simulink model "Car_with_active_suspension_controller"  (R2024b)
settings: Solver=ode45  StartTime=0  StopTime=45  FixedStep=0.001  RelTol=1e-3  AbsTol=1e-6
libraries: simulink_extras x4, Solver_SF x1
settings Model: Creator=ywata  LastModifiedBy=ASUS
settings SolverCC: AutoScaleAbsTol=off  AlgebraicLoopSolver=TrustRegion
settings DataIOCC: SaveFormat=Array  SignalLoggingSaveFormat=ModelDataLogs  ReturnWorkspaceOutputs=off  SignalLoggingName=sigsOut
settings OptimizationCC: BooleanDataType=off  LifeSpan=inf
settings DebuggingCC: SaveWithParameterizedLinksMsg=none  UnderspecifiedInitializationDetection=Classic  MergeDetectMultiDrivingBlocksExec=none  SignalResolutionControl=TryResolveAllWithWarning  MultiTaskDSMMsg=warning  MultiTaskCondExecSysMsg=none  FcnCallInpInsideContextMsg=warning  UnconnectedInputMsg=warning  UnconnectedOutputMsg=warning  UnconnectedLineMsg=warning  StateNameClashWarn=warning  SFUnexpectedBacktrackingDiag=warning  SFNoUnconditionalDefaultTransitionDiag=warning  SFExecutionAtInitializationDiag=none  ArithmeticOperatorsInVariantConditions=warning
settings HardwareCC: ProdBitPerPointer=32  ProdBitPerSizeT=32  ProdBitPerPtrDiffT=32  ProdLargestAtomicFloat=None  ProdIntDivRoundTo=Undefined  ProdEndianess=Unspecified  ProdWordSize=32  ProdHWDeviceType=32-bit Generic  TargetUnknown=on
settings ModelReferenceCC: PropagateSignalLabelsOutOfModel=off
settings RTWCC: TemplateMakefile=grt_vc.tmf  GPUComputeCapability=3.5
settings CodeAppCC: StateflowObjectComments=on
settings GRTTargetCC: TargetLangStandard=C89/C90 (ANSI)  CombineOutputUpdateFcns=off  GRTInterface=on
settings ConfigComp: CovMetricSettings=dw  CovSaveCumulativeToWorkspaceVar=on  CovSaveSingleToWorkspaceVar=on

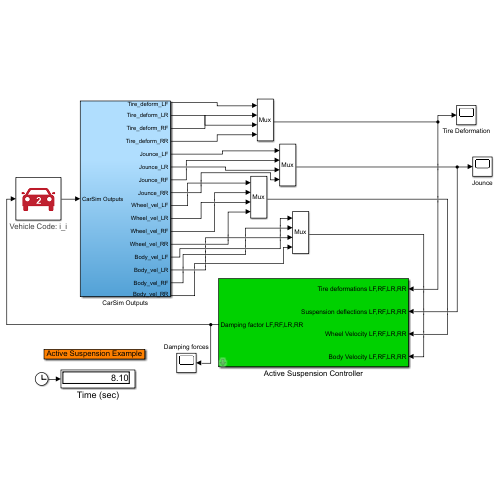
[thumbnail: Simulink's stored preview of the top-level diagram]
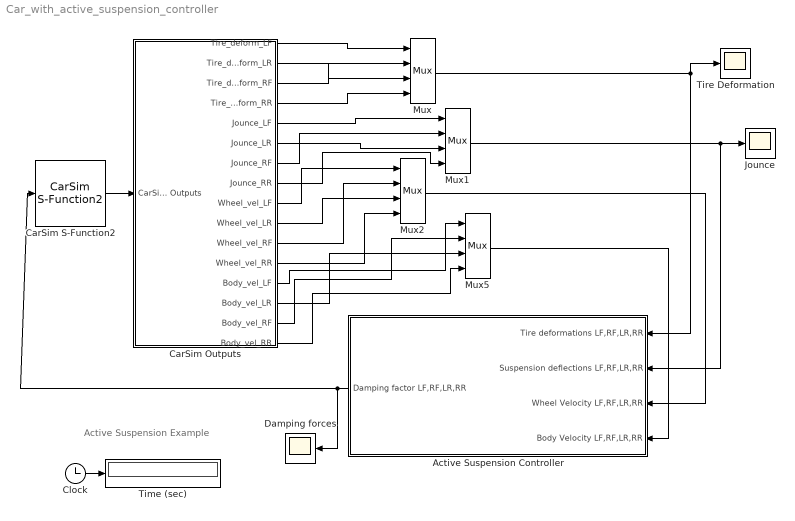
== system Car_with_active_suspension_controller ==
  note: Active Suspension Example
  Active Suspension Controller : Subsystem  mask{K1=-14184, K2=8624, K3=1088, K4=-2504, SP_F=65000, SP_R=52000, GAIN1=1, GAIN2=2.5, UPLIM=40000, LWLIM=10}
      mask prompts: K1 "Optimal control gain, K1"; K2 "Optimal control gain, K2"; K3 "Optimal control gain, K3"; K4 "Optimal control gain, K4"; SP_F "Spring stiffness (front)  (N/m)"; SP_R "Spring stiffness (rear)  (N/m)"; GAIN1 "Gain 1"; GAIN2 "Gain 2"; UPLIM "Variable damper upper limit (N-s/m)"; LWLIM "Variable damper lower limit (N-s/m)"
  CarSim Outputs : Subsystem
  CarSim S-Function2 : Solver_SF/CarSim S-Function2  Priority=1  VehicleCode=i_i  SIMFILE=simfile.sim
      settings: AttributesFormatString=Vehicle Code: %<VehicleCode>  SourceProductName=CarSim S-Function
  Clock : Clock
  Damping forces : Scope
  Jounce : Scope
  Mux{,1..2,5} (4 alike) : Mux
  Time (sec) : Display
      settings: Format=bank  Decimation=100
  Tire Deformation : Scope
  wires:
  Mux2/1 -> Active Suspension Controller/3(Wheel Velocity LF,RF,LR,RR)
  Mux5/1 -> Active Suspension Controller/4(Body Velocity LF,RF,LR,RR)
  Mux/1 -> Active Suspension Controller/1(Tire deformations LF,RF,LR,RR), Tire Deformation/1
  Mux1/1 -> Jounce/1, Active Suspension Controller/2(Suspension deflections LF,RF,LR,RR)
  CarSim Outputs/1(Tire_deform_LF) -> Mux/1
  CarSim Outputs/2(Tire_deform_LR) -> Mux/3
  CarSim Outputs/3(Tire_deform_RF) -> Mux/2
  CarSim Outputs/5(Jounce_LF) -> Mux1/1
  CarSim Outputs/6(Jounce_LR) -> Mux1/3
  CarSim Outputs/7(Jounce_RF) -> Mux1/2
  CarSim Outputs/8(Jounce_RR) -> Mux1/4
  CarSim Outputs/9(Wheel_vel_LF) -> Mux2/1
  CarSim Outputs/10(Wheel_vel_LR) -> Mux2/3
  CarSim Outputs/11(Wheel_vel_RF) -> Mux2/2
  CarSim Outputs/12(Wheel_vel_RR) -> Mux2/4
  CarSim Outputs/13(Body_vel_LF) -> Mux5/1
  CarSim Outputs/14(Body_vel_LR) -> Mux5/3
  CarSim Outputs/15(Body_vel_RF) -> Mux5/2
  CarSim Outputs/16(Body_vel_RR) -> Mux5/4
  CarSim S-Function2/1 -> CarSim Outputs/1(CarSim Outputs)
  CarSim Outputs/4(Tire_deform_RR) -> Mux/4
  Clock/1 -> Time (sec)/1
  Active Suspension Controller/1(Damping factor LF,RF,LR,RR) -> Damping forces/1, CarSim S-Function2/1

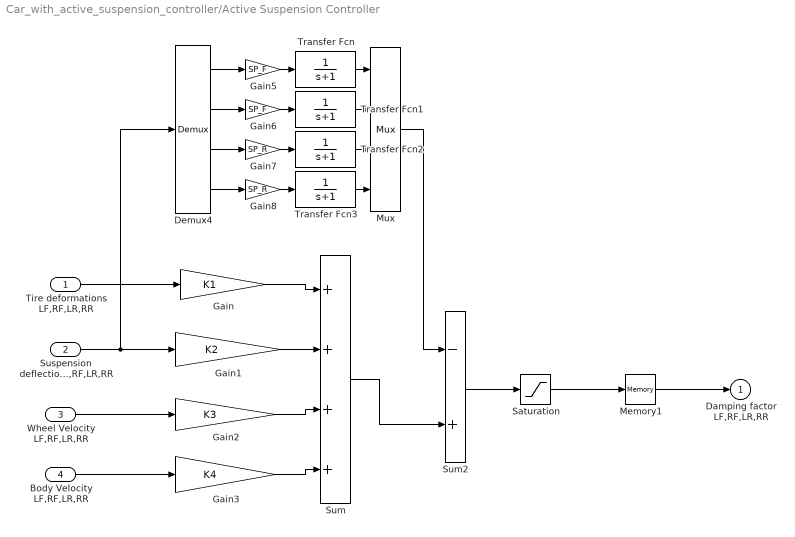
== system Car_with_active_suspension_controller/Active Suspension Controller ==
  Tire deformations LF,RF,LR,RR : Inport
  Suspension deflections LF,RF,LR,RR : Inport  Port=2
  Wheel Velocity LF,RF,LR,RR : Inport  Port=3
  Body Velocity LF,RF,LR,RR : Inport  Port=4
  Demux4 : Demux
      settings: DisplayOption=none
  Gain : Gain  Gain=K1  SaturateOnIntegerOverflow=on  OutDataTypeStr=Inherit: Same as input  ParamDataTypeStr=Inherit: Same as input
  Gain1 : Gain  Gain=K2  SaturateOnIntegerOverflow=on  OutDataTypeStr=Inherit: Same as input  ParamDataTypeStr=Inherit: Same as input
  Gain2 : Gain  Gain=K3  SaturateOnIntegerOverflow=on  OutDataTypeStr=Inherit: Same as input  ParamDataTypeStr=Inherit: Same as input
  Gain3 : Gain  Gain=K4  SaturateOnIntegerOverflow=on  OutDataTypeStr=Inherit: Same as input  ParamDataTypeStr=Inherit: Same as input
  Gain5 : Gain  Gain=SP_F  SaturateOnIntegerOverflow=on  OutDataTypeStr=Inherit: Same as input  ParamDataTypeStr=Inherit: Same as input
  Gain6 : Gain  Gain=SP_F  SaturateOnIntegerOverflow=on  OutDataTypeStr=Inherit: Same as input  ParamDataTypeStr=Inherit: Same as input
  Gain7 : Gain  Gain=SP_R  SaturateOnIntegerOverflow=on  OutDataTypeStr=Inherit: Same as input  ParamDataTypeStr=Inherit: Same as input
  Gain8 : Gain  Gain=SP_R  SaturateOnIntegerOverflow=on  OutDataTypeStr=Inherit: Same as input  ParamDataTypeStr=Inherit: Same as input
  Memory1 : Memory
  Mux : Mux
  Saturation : Saturate  UpperLimit=UPLIM  LowerLimit=LWLIM
  Sum : Sum  Inputs=++++  InputSameDT=on  SaturateOnIntegerOverflow=on  OutDataTypeStr=Inherit: Same as first input
  Sum2 : Sum  Inputs=-+  InputSameDT=on  SaturateOnIntegerOverflow=on  OutDataTypeStr=Inherit: Same as first input
  Transfer Fcn{,1..3} (4 alike) : TransferFcn  Denominator=[1 1]
  Damping factor LF,RF,LR,RR : Outport  InitialOutput=0
  wires:
  Tire deformations LF,RF,LR,RR/1 -> Gain/1
  Gain/1 -> Sum/1
  Gain1/1 -> Sum/2
  Gain2/1 -> Sum/3
  Gain3/1 -> Sum/4
  Sum2/1 -> Saturation/1
  Body Velocity LF,RF,LR,RR/1 -> Gain3/1
  Wheel Velocity LF,RF,LR,RR/1 -> Gain2/1
  Saturation/1 -> Memory1/1
  Memory1/1 -> Damping factor LF,RF,LR,RR/1
  Suspension deflections LF,RF,LR,RR/1 -> Gain1/1, Demux4/1
  Demux4/1 -> Gain5/1
  Demux4/2 -> Gain6/1
  Demux4/3 -> Gain7/1
  Demux4/4 -> Gain8/1
  Sum/1 -> Sum2/2
  Mux/1 -> Sum2/1
  Gain8/1 -> Transfer Fcn3/1
  Transfer Fcn3/1 -> Mux/4
  Gain7/1 -> Transfer Fcn2/1
  Transfer Fcn2/1 -> Mux/3
  Gain6/1 -> Transfer Fcn1/1
  Transfer Fcn1/1 -> Mux/2
  Gain5/1 -> Transfer Fcn/1
  Transfer Fcn/1 -> Mux/1

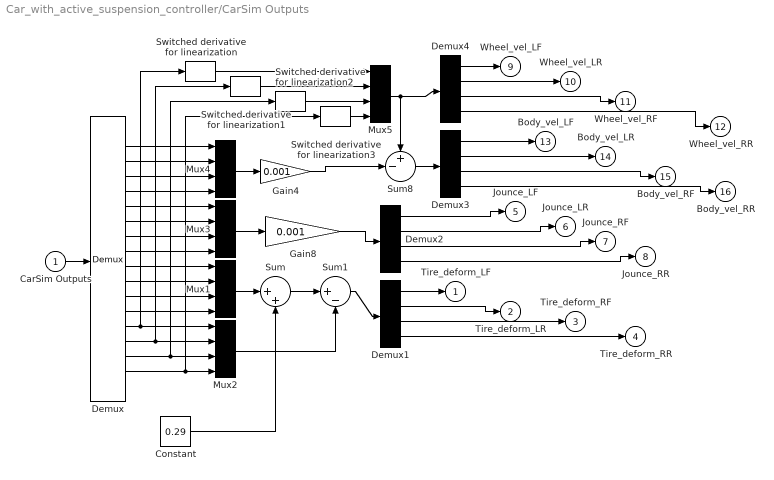
== system Car_with_active_suspension_controller/CarSim Outputs ==
  CarSim Outputs : Inport
  Constant : Constant  Value=0.29
  Demux : Demux  Outputs=16
      settings: DisplayOption=none
  Demux{1..4} (4 alike) : Demux
      settings: DisplayOption=none
  Gain4 : Gain  Gain=0.001  SaturateOnIntegerOverflow=on  OutDataTypeStr=Inherit: Same as input  ParamDataTypeStr=Inherit: Same as input
  Gain8 : Gain  Gain=0.001  SaturateOnIntegerOverflow=on  OutDataTypeStr=Inherit: Same as input  ParamDataTypeStr=Inherit: Same as input
  Mux{1..5} (5 alike) : Mux
  Sum : Sum  Inputs=|++  InputSameDT=on  SaturateOnIntegerOverflow=on  OutDataTypeStr=Inherit: Same as first input
  Sum1 : Sum  Inputs=|+-  InputSameDT=on  SaturateOnIntegerOverflow=on  OutDataTypeStr=Inherit: Same as first input
  Sum8 : Sum  Inputs=+-|  InputSameDT=on  SaturateOnIntegerOverflow=on  OutDataTypeStr=Inherit: Same as first input
  Switched derivative for linearization{,1..3} (4 alike) : simulink_extras/Linearization/Switched derivative for linearization  switchVal=0  derivConst=100
  Tire_deform_LF : Outport  InitialOutput=0
  Tire_deform_LR : Outport  Port=2  InitialOutput=0
  Tire_deform_RF : Outport  Port=3  InitialOutput=0
  Tire_deform_RR : Outport  Port=4  InitialOutput=0
  Jounce_LF : Outport  Port=5  InitialOutput=0
  Jounce_LR : Outport  Port=6  InitialOutput=0
  Jounce_RF : Outport  Port=7  InitialOutput=0
  Jounce_RR : Outport  Port=8  InitialOutput=0
  Wheel_vel_LF : Outport  Port=9  InitialOutput=0
  Wheel_vel_LR : Outport  Port=10  InitialOutput=0
  Wheel_vel_RF : Outport  Port=11  InitialOutput=0
  Wheel_vel_RR : Outport  Port=12  InitialOutput=0
  Body_vel_LF : Outport  Port=13  InitialOutput=0
  Body_vel_LR : Outport  Port=14  InitialOutput=0
  Body_vel_RF : Outport  Port=15  InitialOutput=0
  Body_vel_RR : Outport  Port=16  InitialOutput=0
  wires:
  Sum/1 -> Sum1/1
  Mux1/1 -> Sum/1
  Constant/1 -> Sum/2
  Mux2/1 -> Sum1/2
  Sum1/1 -> Demux1/1
  Demux1/1 -> Tire_deform_LF/1
  Demux1/2 -> Tire_deform_LR/1
  Demux1/3 -> Tire_deform_RF/1
  Demux1/4 -> Tire_deform_RR/1
  Mux3/1 -> Gain8/1
  Gain8/1 -> Demux2/1
  Demux2/1 -> Jounce_LF/1
  Demux2/2 -> Jounce_LR/1
  Demux2/3 -> Jounce_RF/1
  Demux2/4 -> Jounce_RR/1
  Sum8/1 -> Demux3/1
  Demux3/1 -> Body_vel_LF/1
  Demux3/2 -> Body_vel_LR/1
  Demux3/3 -> Body_vel_RF/1
  Demux3/4 -> Body_vel_RR/1
  Demux4/1 -> Wheel_vel_LF/1
  Demux4/2 -> Wheel_vel_LR/1
  Demux4/3 -> Wheel_vel_RF/1
  Demux4/4 -> Wheel_vel_RR/1
  Mux4/1 -> Gain4/1
  Gain4/1 -> Sum8/2
  Demux/12 -> Mux1/4
  Demux/11 -> Mux1/3
  Demux/10 -> Mux1/2
  Demux/9 -> Mux1/1
  Demux/8 -> Mux3/4
  Demux/7 -> Mux3/3
  Demux/6 -> Mux3/2
  Demux/5 -> Mux3/1
  Demux/4 -> Mux4/4
  Demux/3 -> Mux4/3
  Demux/2 -> Mux4/2
  Demux/1 -> Mux4/1
  Demux/13 -> Mux2/1, Switched derivative for linearization/1
  Demux/14 -> Mux2/2, Switched derivative for linearization1/1
  Demux/15 -> Mux2/3, Switched derivative for linearization2/1
  Demux/16 -> Mux2/4, Switched derivative for linearization3/1
  Switched derivative for linearization3/1 -> Mux5/4
  Switched derivative for linearization2/1 -> Mux5/3
  Switched derivative for linearization1/1 -> Mux5/2
  Switched derivative for linearization/1 -> Mux5/1
  Mux5/1 -> Demux4/1, Sum8/1
  CarSim Outputs/1 -> Demux/1
